simulink model "RoboticsCourseworkSimulink1"  (R2021b)
settings: Solver=VariableStepAuto  StartTime=0.0  StopTime=20  RelTol=1e-3
values from neighbouring files (symbols this model uses):
  g = 0    [RoboticsCoursework.m]    (also in matlab.mat)
  k1cg = sqrt(L1/12)    [RoboticsCoursework.m]    (also in matlab.mat = 0.288675134595)
  k2cg = sqrt(L2/12)    [RoboticsCoursework.m]    (also in matlab.mat = 0.288675134595)
  L1 = 1    [RoboticsCoursework.m]    (also in matlab.mat)
  L1cg = 1/2    (= 0.5)    [RoboticsCoursework.m]    (also in matlab.mat)
  L2 = 1    [RoboticsCoursework.m]    (also in matlab.mat)
  L2cg = 1/2    (= 0.5)    [RoboticsCoursework.m]    (also in matlab.mat)
  m = m1    (= 1)    [RoboticsCoursework.m]    (also in matlab.mat)
  m1 = 1    [RoboticsCoursework.m]    (also in matlab.mat)
  m2 = 1    [RoboticsCoursework.m]    (also in matlab.mat)
  mu = mu2    (= 0.1)    [RoboticsCoursework.m]    (also in matlab.mat)
  mu1 = 0.1    [RoboticsCoursework.m]    (also in matlab.mat)
  tou1 = 1    [RoboticsCoursework.m]    (also in matlab.mat)
  tou2 = 1    [RoboticsCoursework.m]    (also in matlab.mat)
  Wn1 = 1    [RoboticsCoursework.m]    (also in matlab.mat)
settings Model: Creator=mic_1  LastModifiedBy=mic_1
settings DataIOCC: ReturnWorkspaceOutputs=off

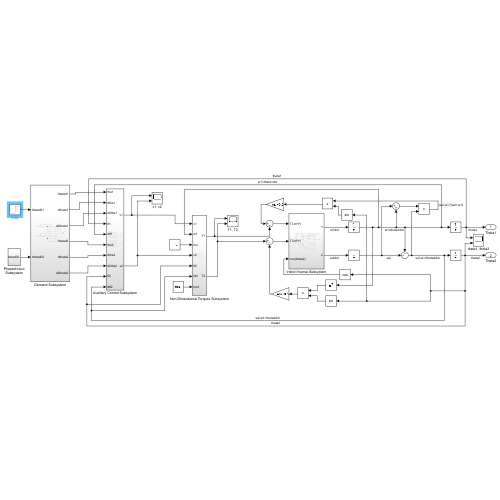
[thumbnail: Simulink's stored preview of the top-level diagram]
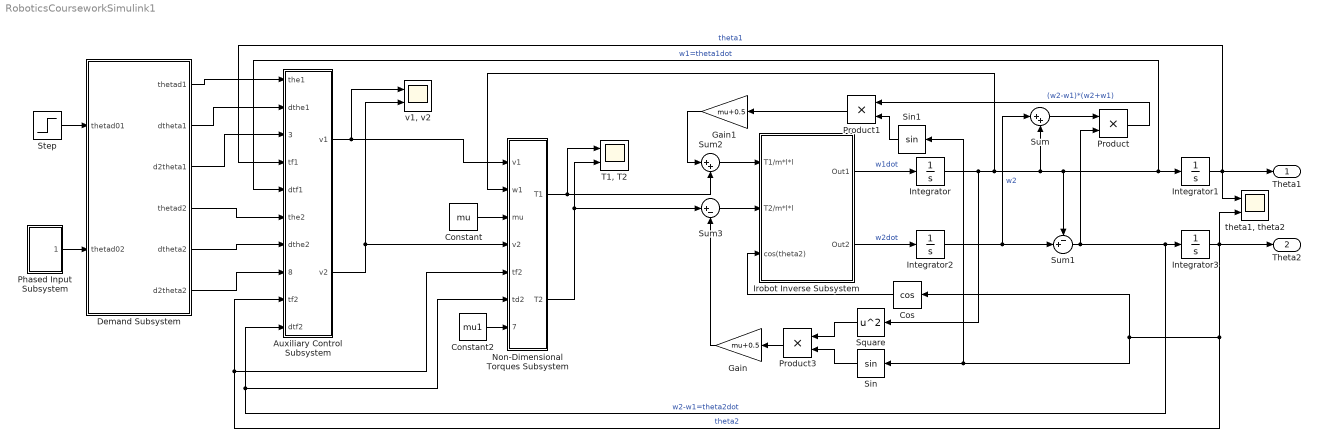
== system RoboticsCourseworkSimulink1 ==
  Auxiliary Control Subsystem : Subsystem
  Constant : Constant  Value=mu
  Constant2 : Constant  Value=mu1
  Cos : Trigonometry  Operator=cos
  Demand Subsystem : Subsystem
  Gain : Gain  Gain=mu+0.5
  Gain1 : Gain  Gain=mu+0.5
  Integrator{,1..3} (4 alike) : Integrator
  Irobot Inverse Subsystem : Subsystem
  Non-Dimensional Torques Subsystem : Subsystem
  Phased Input Subsystem : Subsystem
  Product : Product
  Product1 : Product
  Product3 : Product
  Sin : Trigonometry
  Sin1 : Trigonometry
  Square : Math  Operator=square  SaturateOnIntegerOverflow=on
  Step : Step  After=6.87*pi/180  SampleTime=0
  Sum : Sum  Inputs=|++
  Sum1 : Sum  Inputs=-+|
  Sum2 : Sum  Inputs=|++
  Sum3 : Sum  Inputs=|+-
  "T1, T2" : Scope  NumInputPorts=2
  "theta1, theta2" : Scope  NumInputPorts=2
  "v1, v2" : Scope  NumInputPorts=2
  Theta1 : Outport
  Theta2 : Outport  Port=2
  wires:
  Integrator/1 -> Non-Dimensional Torques Subsystem/2(w1), Auxiliary Control Subsystem/5(dtf1), Integrator1/1, Sum1/1, Sum/2, Square/1  "w1=theta1dot"
  Sum/1 -> Product/1
  Integrator2/1 -> Sum/1, Sum1/2  "w2"
  Sum1/1 -> Product/2, Auxiliary Control Subsystem/10(dtf2), Non-Dimensional Torques Subsystem/6(td2), Integrator3/1  "w2-w1=theta2dot"
  Integrator1/1 -> "theta1, theta2"/1, Theta1/1, Auxiliary Control Subsystem/4(tf1)  "theta1"
  Square/1 -> Product3/1
  Sin/1 -> Product3/2
  Product3/1 -> Gain/1
  Integrator3/1 -> Theta2/1, Non-Dimensional Torques Subsystem/5(tf2), Auxiliary Control Subsystem/9(tf2), Sin1/1, Sin/1, Cos/1, "theta1, theta2"/2  "theta2"
  Product/1 -> Product1/1  "(w2-w1)*(w2+w1)"
  Sin1/1 -> Product1/2
  Product1/1 -> Gain1/1
  Gain1/1 -> Sum2/1
  Gain/1 -> Sum3/2
  Irobot Inverse Subsystem/1(Out1) -> Integrator/1  "w1dot"
  Irobot Inverse Subsystem/2(Out2) -> Integrator2/1  "w2dot"
  Cos/1 -> Irobot Inverse Subsystem/3(cos(theta2))
  Sum3/1 -> Irobot Inverse Subsystem/2(T2/m*l*l)
  Sum2/1 -> Irobot Inverse Subsystem/1(T1/m*l*l)
  Auxiliary Control Subsystem/1(v1) -> Non-Dimensional Torques Subsystem/1(v1), "v1, v2"/1
  Auxiliary Control Subsystem/2(v2) -> Non-Dimensional Torques Subsystem/4(v2), "v1, v2"/2
  Demand Subsystem/1(thetad1) -> Auxiliary Control Subsystem/1(the1)
  Demand Subsystem/2(dtheta1) -> Auxiliary Control Subsystem/2(dthe1)
  Demand Subsystem/3(d2theta1) -> Auxiliary Control Subsystem/3(d2the1)
  Step/1 -> Demand Subsystem/1(thetad01)
  Demand Subsystem/4(thetad2) -> Auxiliary Control Subsystem/6(the2)
  Demand Subsystem/6(d2theta2) -> Auxiliary Control Subsystem/8(d2the2)
  Demand Subsystem/5(dtheta2) -> Auxiliary Control Subsystem/7(dthe2)
  Non-Dimensional Torques Subsystem/1(T1) -> Sum2/2, "T1, T2"/1
  Non-Dimensional Torques Subsystem/2(T2) -> Sum3/1, "T1, T2"/2
  Constant/1 -> Non-Dimensional Torques Subsystem/3(mu)
  Constant2/1 -> Non-Dimensional Torques Subsystem/7(mu1)
  Phased Input Subsystem/1(thetad02) -> Demand Subsystem/2(thetad02)

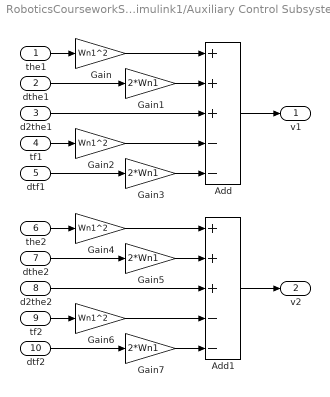
== system RoboticsCourseworkSimulink1/Auxiliary Control Subsystem ==
  the1 : Inport
  dthe1 : Inport  Port=2
  d2the1 : Inport  Port=3
  tf1 : Inport  Port=4
  dtf1 : Inport  Port=5
  the2 : Inport  Port=6
  dthe2 : Inport  Port=7
  d2the2 : Inport  Port=8
  tf2 : Inport  Port=9
  dtf2 : Inport  Port=10
  Add : Sum  Inputs=+++--
  Add1 : Sum  Inputs=+++--
  Gain{,2,4,6} (4 alike) : Gain  Gain=Wn1^2
  Gain{1,3,5,7} (4 alike) : Gain  Gain=2*Wn1
  v1 : Outport
  v2 : Outport  Port=2
  wires:
  Add/1 -> v1/1
  Gain/1 -> Add/1
  d2the1/1 -> Add/3
  Gain2/1 -> Add/4
  the1/1 -> Gain/1
  Gain1/1 -> Add/2
  dthe1/1 -> Gain1/1
  tf1/1 -> Gain2/1
  Gain3/1 -> Add/5
  dtf1/1 -> Gain3/1
  tf2/1 -> Gain6/1
  Gain4/1 -> Add1/1
  Gain5/1 -> Add1/2
  the2/1 -> Gain4/1
  dthe2/1 -> Gain5/1
  dtf2/1 -> Gain7/1
  Gain7/1 -> Add1/5
  Add1/1 -> v2/1
  Gain6/1 -> Add1/4
  d2the2/1 -> Add1/3

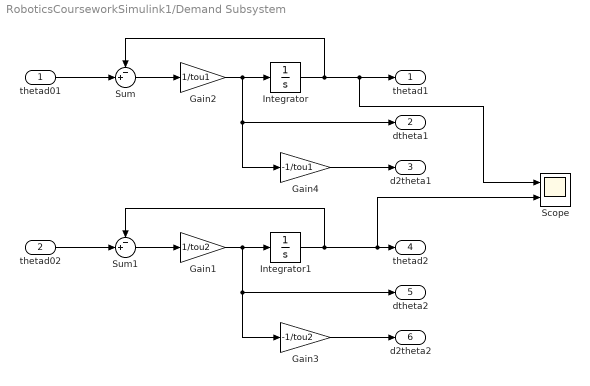
== system RoboticsCourseworkSimulink1/Demand Subsystem ==
  thetad01 : Inport
  thetad02 : Inport  Port=2
  Gain1 : Gain  Gain=1/tou2
  Gain2 : Gain  Gain=1/tou1
  Gain3 : Gain  Gain=-1/tou2
  Gain4 : Gain  Gain=-1/tou1
  Integrator : Integrator
  Integrator1 : Integrator
  Scope : Scope  NumInputPorts=2
  Sum : Sum  Inputs=-+|
  Sum1 : Sum  Inputs=-+|
  thetad1 : Outport
  dtheta1 : Outport  Port=2
  d2theta1 : Outport  Port=3
  thetad2 : Outport  Port=4
  dtheta2 : Outport  Port=5
  d2theta2 : Outport  Port=6
  wires:
  thetad01/1 -> Sum/2
  Sum/1 -> Gain2/1
  Gain2/1 -> dtheta1/1, Gain4/1, Integrator/1
  Integrator/1 -> Scope/1, thetad1/1, Sum/1
  Gain4/1 -> d2theta1/1
  Integrator1/1 -> Scope/2, thetad2/1, Sum1/1
  Gain3/1 -> d2theta2/1
  Gain1/1 -> dtheta2/1, Gain3/1, Integrator1/1
  Sum1/1 -> Gain1/1
  thetad02/1 -> Sum1/2

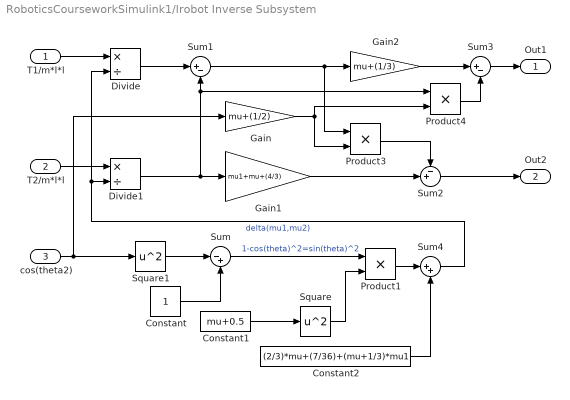
== system RoboticsCourseworkSimulink1/Irobot Inverse Subsystem ==
  T1/m*l*l : Inport
  T2/m*l*l : Inport  Port=2
  cos(theta2) : Inport  Port=3
  Constant : Constant
  Constant1 : Constant  Value=mu+0.5
  Constant2 : Constant  Value=(2/3)*mu+(7/36)+(mu+1/3)*mu1
  Divide : Product  Inputs=*/
  Divide1 : Product  Inputs=*/
  Gain : Gain  Gain=mu+(1/2)
  Gain1 : Gain  Gain=mu1+mu+(4/3)
  Gain2 : Gain  Gain=mu+(1/3)
  Product1 : Product
  Product3 : Product
  Product4 : Product
  Square : Math  Operator=square  SaturateOnIntegerOverflow=on
  Square1 : Math  Operator=square  SaturateOnIntegerOverflow=on
  Sum : Sum  Inputs=|-+
  Sum1 : Sum  Inputs=|+-
  Sum2 : Sum  Inputs=-+|
  Sum3 : Sum  Inputs=|+-
  Sum4 : Sum  Inputs=|++
  Out1 : Outport
  Out2 : Outport  Port=2
  wires:
  T1/m*l*l/1 -> Divide/1
  T2/m*l*l/1 -> Divide1/1
  cos(theta2)/1 -> Square1/1, Gain/1
  Divide/1 -> Sum1/1
  Divide1/1 -> Product4/1, Sum1/2, Gain1/1
  Constant/1 -> Sum/2
  Sum1/1 -> Product3/1, Gain2/1
  Gain2/1 -> Sum3/1
  Product4/1 -> Sum3/2
  Gain/1 -> Product3/2, Product4/2
  Sum3/1 -> Out1/1
  Sum2/1 -> Out2/1
  Sum4/1 -> Divide/2, Divide1/2  "delta(mu1,mu2)"
  Product1/1 -> Sum4/1
  Square/1 -> Product1/2
  Sum/1 -> Product1/1  "1-cos(theta)^2=sin(theta)^2"
  Constant2/1 -> Sum4/2
  Constant1/1 -> Square/1
  Square1/1 -> Sum/1
  Gain1/1 -> Sum2/2
  Product3/1 -> Sum2/1

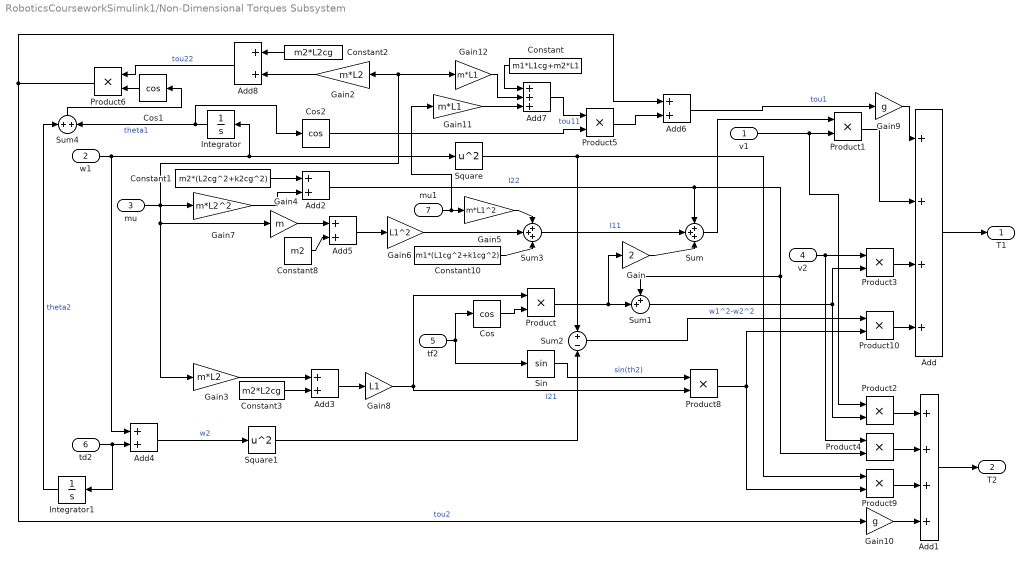
== system RoboticsCourseworkSimulink1/Non-Dimensional Torques Subsystem ==
  v1 : Inport
  w1 : Inport  Port=2
  mu : Inport  Port=3
  v2 : Inport  Port=4
  tf2 : Inport  Port=5
  td2 : Inport  Port=6
  mu1 : Inport  Port=7
  Add : Sum  Inputs=++++
  Add1 : Sum  Inputs=++++
  Add{2..6,8} (6 alike) : Sum
  Add7 : Sum  Inputs=+++
  Constant : Constant  Value=m1*L1cg+m2*L1
  Constant1 : Constant  Value=m2*(L2cg^2+k2cg^2)
  Constant10 : Constant  Value=m1*(L1cg^2+k1cg^2)
  Constant2 : Constant  Value=m2*L2cg
  Constant3 : Constant  Value=m2*L2cg
  Constant8 : Constant  Value=m2
  Cos : Trigonometry  Operator=cos
  Cos1 : Trigonometry  Operator=cos
  Cos2 : Trigonometry  Operator=cos
  Gain : Gain  Gain=2
  Gain10 : Gain  Gain=g
  Gain11 : Gain  Gain=m*L1
  Gain12 : Gain  Gain=m*L1
  Gain2 : Gain  Gain=m*L2
  Gain3 : Gain  Gain=m*L2
  Gain4 : Gain  Gain=m
  Gain5 : Gain  Gain=m*L1^2
  Gain6 : Gain  Gain=L1^2
  Gain7 : Gain  Gain=m*L2^2
  Gain8 : Gain  Gain=L1
  Gain9 : Gain  Gain=g
  Integrator : Integrator
  Integrator1 : Integrator
  Product{,1..6,8..10} (10 alike) : Product
  Sin : Trigonometry
  Square : Math  Operator=square  SaturateOnIntegerOverflow=on
  Square1 : Math  Operator=square  SaturateOnIntegerOverflow=on
  Sum : Sum  Inputs=+++
  Sum1 : Sum  Inputs=++|
  Sum2 : Sum  Inputs=+-
  Sum3 : Sum  Inputs=+++
  Sum4 : Sum
  T1 : Outport
  T2 : Outport  Port=2
  wires:
  tf2/1 -> Cos/1, Sin/1
  Cos/1 -> Product/2
  Sum/1 -> Product1/1
  v1/1 -> Product2/1, Product1/2
  Product1/1 -> Add/2
  Product/1 -> Gain/1, Sum1/2
  Sum1/1 -> Product3/2, Product2/2
  v2/1 -> Product4/1, Product3/1
  Product3/1 -> Add/3
  Product2/1 -> Add1/1
  Product4/1 -> Add1/2
  mu/1 -> Gain12/1, Gain2/1, Gain3/1, Gain4/1, Gain7/1
  Constant1/1 -> Add2/1
  Add2/1 -> Product4/2, Sum1/1, Sum/1  "I22"
  Gain3/1 -> Add3/1
  Constant3/1 -> Add3/2
  Add3/1 -> Gain8/1
  Gain8/1 -> Product8/2, Product/1  "I21"
  Gain10/1 -> Add1/4
  Add/1 -> T1/1
  Add1/1 -> T2/1
  w1/1 -> Add4/1, Square/1, Integrator/1
  Sin/1 -> Product8/1  "sin(th2)"
  Product8/1 -> Product10/2, Product9/2
  Square/1 -> Sum2/1, Product9/1
  Product9/1 -> Add1/3
  td2/1 -> Add4/2, Integrator1/1
  Add4/1 -> Square1/1  "w2"
  Square1/1 -> Sum2/2
  Sum2/1 -> Product10/1  "w1^2-w2^2"
  Product10/1 -> Add/4
  Constant8/1 -> Add5/2
  Gain4/1 -> Add5/1
  Constant10/1 -> Sum3/3
  mu1/1 -> Gain11/1, Gain5/1
  Integrator/1 -> Sum4/2, Cos2/1  "theta1"
  Integrator1/1 -> Sum4/1  "theta2"
  Sum4/1 -> Cos1/1
  Product6/1 -> Add6/1, Gain10/1  "tou2"
  Gain9/1 -> Add/1
  Add5/1 -> Gain6/1
  Gain7/1 -> Add2/2
  Add6/1 -> Gain9/1  "tou1"
  Gain/1 -> Sum/3
  Sum3/1 -> Sum/2  "I11"
  Gain5/1 -> Sum3/1
  Gain6/1 -> Sum3/2
  Gain11/1 -> Add7/3
  Gain12/1 -> Add7/2
  Add7/1 -> Product5/1  "tou11"
  Cos2/1 -> Product5/2
  Product5/1 -> Add6/2
  Constant/1 -> Add7/1
  Gain2/1 -> Add8/2
  Constant2/1 -> Add8/1
  Add8/1 -> Product6/1  "tou22"
  Cos1/1 -> Product6/2

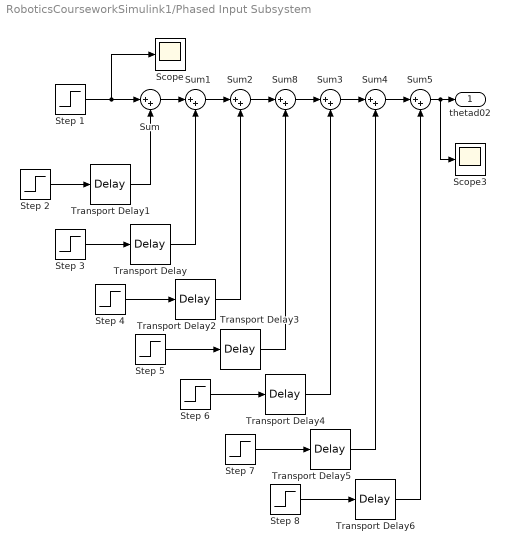
== system RoboticsCourseworkSimulink1/Phased Input Subsystem ==
  Scope : Scope
  Scope3 : Scope
  Step {1..8} (8 alike) : Step  After=30*pi/180  SampleTime=0
  Sum{,1..5,8} (7 alike) : Sum  Inputs=|++
  Transport Delay : TransportDelay  DelayTime=2
  Transport Delay1 : TransportDelay
  Transport Delay2 : TransportDelay  DelayTime=3
  Transport Delay3 : TransportDelay  DelayTime=4
  Transport Delay4 : TransportDelay  DelayTime=5
  Transport Delay5 : TransportDelay  DelayTime=6
  Transport Delay6 : TransportDelay  DelayTime=7
  thetad02 : Outport
  wires:
  Sum/1 -> Sum1/1
  Step 1/1 -> Scope/1, Sum/1
  Step 2/1 -> Transport Delay1/1
  Transport Delay1/1 -> Sum/2
  Step 3/1 -> Transport Delay/1
  Transport Delay/1 -> Sum1/2
  Transport Delay2/1 -> Sum2/2
  Step 4/1 -> Transport Delay2/1
  Sum1/1 -> Sum2/1
  Step 5/1 -> Transport Delay3/1
  Transport Delay3/1 -> Sum8/2
  Step 6/1 -> Transport Delay4/1
  Step 7/1 -> Transport Delay5/1
  Transport Delay5/1 -> Sum4/2
  Sum2/1 -> Sum8/1
  Step 8/1 -> Transport Delay6/1
  Transport Delay6/1 -> Sum5/2
  Transport Delay4/1 -> Sum3/2
  Sum8/1 -> Sum3/1
  Sum3/1 -> Sum4/1
  Sum4/1 -> Sum5/1
  Sum5/1 -> Scope3/1, thetad02/1
